simulink model "QBot2e_Forward_Kinematics"  (Simulink 8.9)
settings: Solver=ode1  StartTime=0.0  StopTime=inf  FixedStep=0.01  RelTol=1e-3  EnableMultiTasking=on
undefined symbols (not defined in the file or in its folder): HIL
libraries: quarc_library x7
settings Model: Creator=rhuq  LastModifiedBy=amolki  SimulationMode=external  ExtModeTrigDuration=10000
settings SolverCC: PositivePriorityOrder=on
settings OptimizationCC: ExpressionDepthLimit=2147483647  InitFltsAndDblsToZero=on  LifeSpan=auto
settings DebuggingCC: SaveWithParameterizedLinksMsg=none  SolverPrmCheckMsg=warning  ParameterPrecisionLossMsg=none
settings SFSimCC: SimParseCustomCode=off
settings RTWCC: SystemTargetFile=quarc_linux_pi_3.tlc  TemplateMakefile=quarc_linux_pi_3_tmf  Description=QUARC Linux Raspberry Pi 3 Target
settings STFCustomTargetCC: TargetLibSuffix=.a  TargetPreCompLibLocation=C:\PROGRA~3\QUARC\lib\2017a\LICFC8~1\release  ConcurrentExecutionCompliant=on  SystemTargetFile=quarc_linux_pi_3.tlc
settings GRTTargetCC: TargetLibSuffix=.a  TargetPreCompLibLocation=C:\PROGRA~3\QUARC\lib\2017a\LICFC8~1\release  ParMdlRefBuildCompliant=off  CompOptLevelCompliant=off  GeneratePreprocessorConditionals=Use local settings  MatFileLogging=off  CPPClassGenCompliant=off  UseToolchainInfoCompliant=off  ExtMode=on  ExtModeMexFile=quarc_comm  ExtModeMexArgs='-w -d /tmp -uri %u'

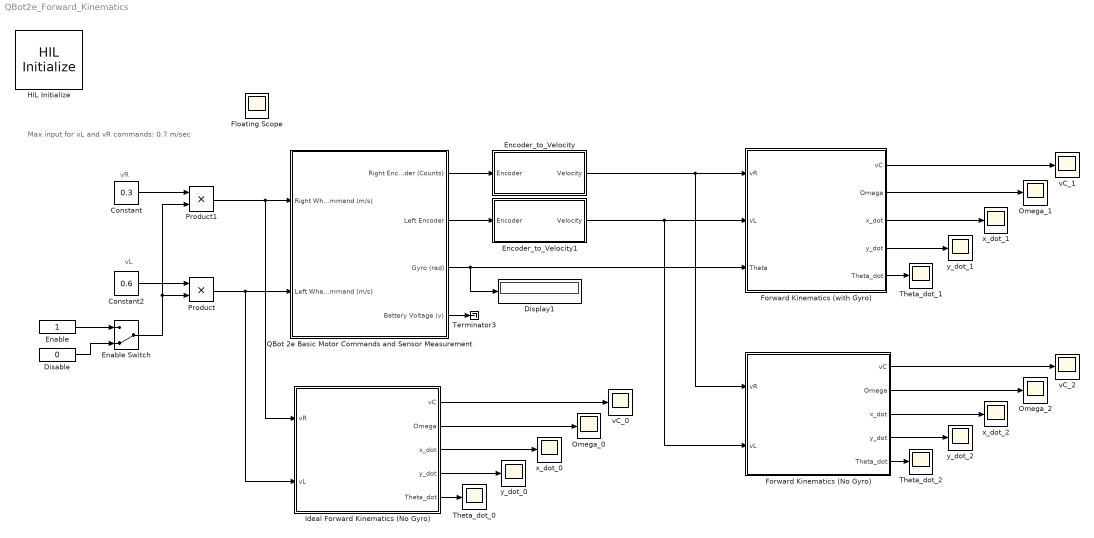
== system QBot2e_Forward_Kinematics ==
  note: vL
  note: vR
  note: Max input for vL and vR commands: 0.7 m/sec
  Constant : Constant  Value=0.3
  Constant2 : Constant  Value=0.6
  Disable : Constant  Value=0
  Display1 : Display
  Enable : Constant
  Enable Switch : ManualSwitch  CurrentSetting=0
  Encoder_to_Velocity : Subsystem
  Encoder_to_Velocity1 : Subsystem
  Forward Kinematics (No Gyro) : Subsystem
  Forward Kinematics (with Gyro) : Subsystem
  HIL Initialize : quarc_library/Data Acquisition/Generic/Configuration/HIL Initialize  Priority=-99  object_name=HIL-1  board_type=qbot2e  board_number=0  board_options=pwm0_en=1;pwm0_pin=12;pwm1_en=1;pwm1_pin=13;  exclusive=off  active=off  hardware_clocks=[]  clock_modes=[]  initial_clock_frequencies=[]  set_clock_params_at_start=off  set_clock_params_at_switch_in=off  set_clock_frequencies_at_start=off  set_clock_frequencies_at_switch_in=off  analog_input_channels=[0:5]  analog_input_configurations=[]  analog_input_maximums=[16.5 3.3 3.3 3.3 3.3 3.3]  analog_input_minimums=[0 0 0 0 0 0]  set_analog_input_params_at_start=off  set_analog_input_params_at_switch_in=off  analog_output_channels=[]  analog_output_maximums=[]  analog_output_minimums=[]  initial_analog_outputs=[]  final_analog_outputs=[]  watchdog_analog_outputs=[]  set_analog_output_params_at_start=off  set_analog_output_params_at_switch_in=off  set_analog_outputs_at_start=off  set_analog_outputs_at_switch_in=off  set_analog_outputs_at_terminate=off  set_analog_outputs_at_switch_out=off  set_analog_outputs_on_watchdog=off  digital_input_channels=[28:58]  digital_output_channels=[28:31]  digital_output_configuration=[]  initial_digital_outputs=[0]  final_digital_outputs=[0]  watchdog_digital_outputs=[]  set_digital_output_params_at_start=off  set_digital_output_params_at_switch_in=off  set_digital_outputs_at_start=on  set_digital_outputs_at_switch_in=off  set_digital_outputs_at_terminate=on  set_digital_outputs_at_switch_out=off  set_digital_outputs_on_watchdog=off  encoder_channels=[0:1]  quadrature=[4]  encoder_filter_frequency=[]  initial_encoder_counts=[0]  set_encoder_params_at_start=on  set_encoder_params_at_switch_in=off  set_encoder_counts_at_start=on  set_encoder_counts_at_switch_in=off  pwm_channels=[0:1]  pwm_modes=0  pwm_frequency=100e6 / 4095  pwm_configuration=[0]  pwm_alignment=[0]  pwm_polarity=[1]  pwm_leading_deadband=[]  pwm_trailing_deadband=[]  initial_pwm_outputs=[0]  final_pwm_outputs=[0]  watchdog_pwm_outputs=[]  set_pwm_params_at_start=on  set_pwm_params_at_switch_in=off  set_pwm_outputs_at_start=on  set_pwm_outputs_at_switch_in=off  set_pwm_outputs_at_terminate=on  set_pwm_outputs_at_switch_out=off  set_pwm_outputs_on_watchdog=off  other_output_channels=[2000:2001 14000 16000]  initial_other_outputs=[0 0 0 7]  final_other_outputs=[0 0 0 7]  watchdog_other_outputs=[]  set_other_outputs_at_start=on  set_other_outputs_at_switch_in=off  set_other_outputs_at_terminate=on  set_other_outputs_at_switch_out=off  set_other_outputs_on_watchdog=off
  Ideal Forward Kinematics (No Gyro) : Subsystem
  Omega_0 : Scope
  Omega_1 : Scope
  Omega_2 : Scope
  Product : Product  RndMeth=Zero
  Product1 : Product  RndMeth=Zero
  QBot 2e Basic Motor Commands and Sensor Measurement : Subsystem
  Terminator3 : Terminator
  Theta_dot_0 : Scope
  Theta_dot_1 : Scope
  Theta_dot_2 : Scope
  vC_0 : Scope
  vC_1 : Scope
  vC_2 : Scope
  x_dot_0 : Scope
  x_dot_1 : Scope
  x_dot_2 : Scope
  y_dot_0 : Scope
  y_dot_1 : Scope
  y_dot_2 : Scope
  Floating Scope : Scope
  wires:
  QBot 2e Basic Motor Commands and Sensor Measurement/1(Right Encoder (Counts)) -> Encoder_to_Velocity/1(Encoder)
  QBot 2e Basic Motor Commands and Sensor Measurement/2(Left Encoder) -> Encoder_to_Velocity1/1(Encoder)
  QBot 2e Basic Motor Commands and Sensor Measurement/3(Gyro (rad)) -> Display1/1, Forward Kinematics (with Gyro)/3(Theta)
  Encoder_to_Velocity1/1(Velocity) -> Forward Kinematics (No Gyro)/2(vL), Forward Kinematics (with Gyro)/2(vL)
  Ideal Forward Kinematics (No Gyro)/1(vC) -> vC_0/1
  Ideal Forward Kinematics (No Gyro)/2(Omega) -> Omega_0/1
  Encoder_to_Velocity/1(Velocity) -> Forward Kinematics (No Gyro)/1(vR), Forward Kinematics (with Gyro)/1(vR)
  Enable/1 -> Enable Switch/1
  Disable/1 -> Enable Switch/2
  Constant2/1 -> Product/1
  Constant/1 -> Product1/1
  Enable Switch/1 -> Product/2, Product1/2
  Product1/1 -> QBot 2e Basic Motor Commands and Sensor Measurement/1(Right Wheel Command (m/s)), Ideal Forward Kinematics (No Gyro)/1(vR)
  Product/1 -> Ideal Forward Kinematics (No Gyro)/2(vL), QBot 2e Basic Motor Commands and Sensor Measurement/2(Left Wheel Command (m/s))
  Ideal Forward Kinematics (No Gyro)/3(x_dot) -> x_dot_0/1
  Ideal Forward Kinematics (No Gyro)/4(y_dot) -> y_dot_0/1
  Ideal Forward Kinematics (No Gyro)/5(Theta_dot) -> Theta_dot_0/1
  Forward Kinematics (with Gyro)/1(vC) -> vC_1/1
  Forward Kinematics (with Gyro)/2(Omega) -> Omega_1/1
  Forward Kinematics (with Gyro)/3(x_dot) -> x_dot_1/1
  Forward Kinematics (with Gyro)/4(y_dot) -> y_dot_1/1
  Forward Kinematics (with Gyro)/5(Theta_dot) -> Theta_dot_1/1
  Forward Kinematics (No Gyro)/1(vC) -> vC_2/1
  Forward Kinematics (No Gyro)/2(Omega) -> Omega_2/1
  Forward Kinematics (No Gyro)/3(x_dot) -> x_dot_2/1
  Forward Kinematics (No Gyro)/4(y_dot) -> y_dot_2/1
  Forward Kinematics (No Gyro)/5(Theta_dot) -> Theta_dot_2/1
  QBot 2e Basic Motor Commands and Sensor Measurement/4(Battery Voltage (v)) -> Terminator3/1

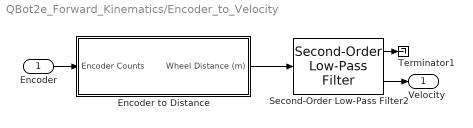
== system QBot2e_Forward_Kinematics/Encoder_to_Velocity ==
  Encoder : Inport
  Encoder to Distance : Subsystem
  Second-Order Low-Pass Filter2 : quarc_library/Continuous/Second-Order Low-Pass Filter  params_source=Internal (dialog parameters)  input_width=10  input_zeta=1  input_init=0
  Terminator1 : Terminator
  Velocity : Outport
  wires:
  Second-Order Low-Pass Filter2/2 -> Velocity/1
  Encoder/1 -> Encoder to Distance/1(Encoder Counts)
  Encoder to Distance/1(Wheel Distance (m)) -> Second-Order Low-Pass Filter2/1
  Second-Order Low-Pass Filter2/1 -> Terminator1/1

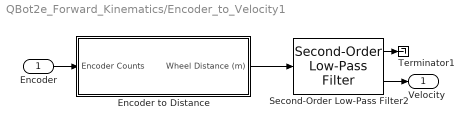
== system QBot2e_Forward_Kinematics/Encoder_to_Velocity1 ==
  Encoder : Inport
  Encoder to Distance : Subsystem
  Second-Order Low-Pass Filter2 : quarc_library/Continuous/Second-Order Low-Pass Filter  params_source=Internal (dialog parameters)  input_width=10  input_zeta=1  input_init=0
  Terminator1 : Terminator
  Velocity : Outport
  wires:
  Second-Order Low-Pass Filter2/2 -> Velocity/1
  Encoder/1 -> Encoder to Distance/1(Encoder Counts)
  Encoder to Distance/1(Wheel Distance (m)) -> Second-Order Low-Pass Filter2/1
  Second-Order Low-Pass Filter2/1 -> Terminator1/1

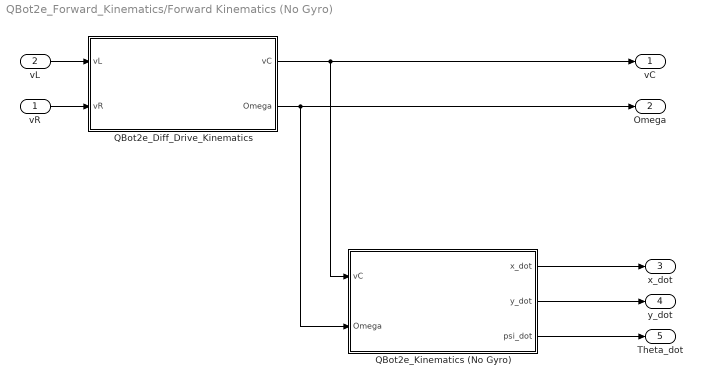
== system QBot2e_Forward_Kinematics/Forward Kinematics (No Gyro) ==
  vR : Inport
  vL : Inport  Port=2
  QBot2e_Diff_Drive_Kinematics : Subsystem
  QBot2e_Kinematics (No Gyro) : Subsystem
  vC : Outport
  Omega : Outport  Port=2
  x_dot : Outport  Port=3
  y_dot : Outport  Port=4
  Theta_dot : Outport  Port=5
  wires:
  QBot2e_Diff_Drive_Kinematics/2(Omega) -> QBot2e_Kinematics (No Gyro)/2(Omega), Omega/1
  vR/1 -> QBot2e_Diff_Drive_Kinematics/2(vR)
  vL/1 -> QBot2e_Diff_Drive_Kinematics/1(vL)
  QBot2e_Diff_Drive_Kinematics/1(vC) -> QBot2e_Kinematics (No Gyro)/1(vC), vC/1
  QBot2e_Kinematics (No Gyro)/2(y_dot) -> y_dot/1
  QBot2e_Kinematics (No Gyro)/1(x_dot) -> x_dot/1
  QBot2e_Kinematics (No Gyro)/3(psi_dot) -> Theta_dot/1

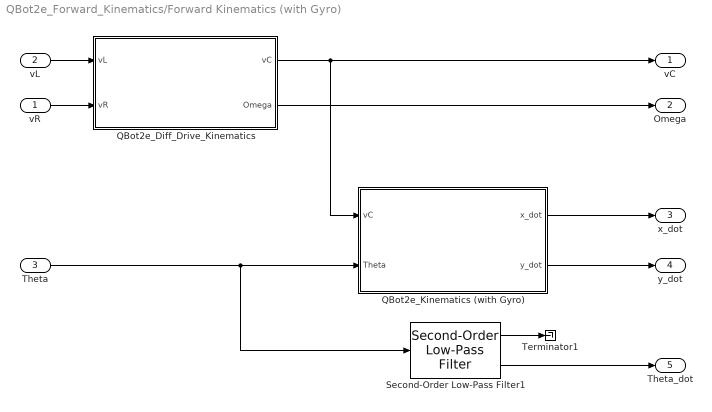
== system QBot2e_Forward_Kinematics/Forward Kinematics (with Gyro) ==
  vR : Inport
  vL : Inport  Port=2
  Theta : Inport  Port=3
  QBot2e_Diff_Drive_Kinematics : Subsystem
  QBot2e_Kinematics (with Gyro) : Subsystem
  Second-Order Low-Pass Filter1 : quarc_library/Continuous/Second-Order Low-Pass Filter  params_source=Internal (dialog parameters)  input_width=60  input_zeta=1  input_init=0
  Terminator1 : Terminator
  vC : Outport
  Omega : Outport  Port=2
  x_dot : Outport  Port=3
  y_dot : Outport  Port=4
  Theta_dot : Outport  Port=5
  wires:
  Second-Order Low-Pass Filter1/2 -> Theta_dot/1
  Second-Order Low-Pass Filter1/1 -> Terminator1/1
  QBot2e_Kinematics (with Gyro)/1(x_dot) -> x_dot/1
  QBot2e_Diff_Drive_Kinematics/1(vC) -> QBot2e_Kinematics (with Gyro)/1(vC), vC/1
  vL/1 -> QBot2e_Diff_Drive_Kinematics/1(vL)
  vR/1 -> QBot2e_Diff_Drive_Kinematics/2(vR)
  QBot2e_Diff_Drive_Kinematics/2(Omega) -> Omega/1
  QBot2e_Kinematics (with Gyro)/2(y_dot) -> y_dot/1
  Theta/1 -> QBot2e_Kinematics (with Gyro)/2(Theta), Second-Order Low-Pass Filter1/1

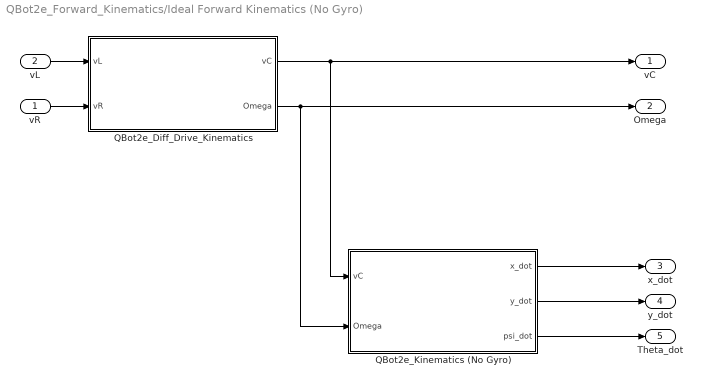
== system QBot2e_Forward_Kinematics/Ideal Forward Kinematics (No Gyro) ==
  vR : Inport
  vL : Inport  Port=2
  QBot2e_Diff_Drive_Kinematics : Subsystem
  QBot2e_Kinematics (No Gyro) : Subsystem
  vC : Outport
  Omega : Outport  Port=2
  x_dot : Outport  Port=3
  y_dot : Outport  Port=4
  Theta_dot : Outport  Port=5
  wires:
  QBot2e_Diff_Drive_Kinematics/2(Omega) -> QBot2e_Kinematics (No Gyro)/2(Omega), Omega/1
  vR/1 -> QBot2e_Diff_Drive_Kinematics/2(vR)
  vL/1 -> QBot2e_Diff_Drive_Kinematics/1(vL)
  QBot2e_Diff_Drive_Kinematics/1(vC) -> QBot2e_Kinematics (No Gyro)/1(vC), vC/1
  QBot2e_Kinematics (No Gyro)/2(y_dot) -> y_dot/1
  QBot2e_Kinematics (No Gyro)/1(x_dot) -> x_dot/1
  QBot2e_Kinematics (No Gyro)/3(psi_dot) -> Theta_dot/1

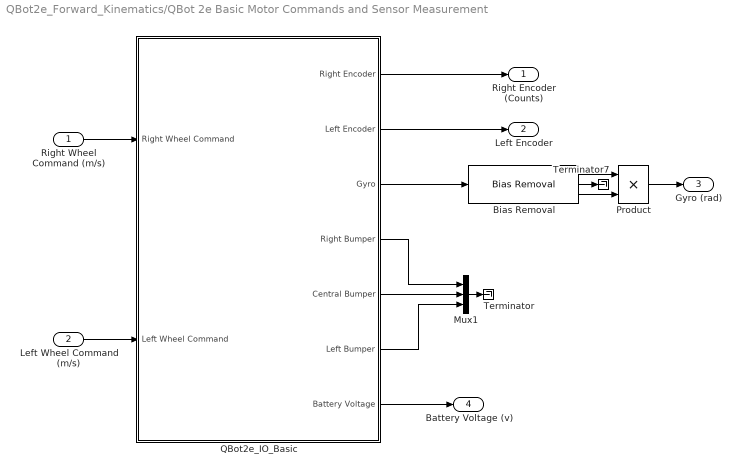
== system QBot2e_Forward_Kinematics/QBot 2e Basic Motor Commands and Sensor Measurement ==
  Right Wheel Command (m/s) : Inport
  Left Wheel Command (m/s) : Inport  Port=2
  Bias Removal : quarc_library/Discrete/Bias Removal  start_time=3  end_time=4  switch_id=0  sample_time=qc_get_step_size
      settings: SourceProductName=QUARC Targets
  Mux1 : Mux  Inputs=3
  Product : Product  RndMeth=Zero
  QBot2e_IO_Basic : Subsystem
  Terminator : Terminator
  Terminator7 : Terminator
  Right Encoder (Counts) : Outport
  Left Encoder : Outport  Port=2
  Gyro (rad) : Outport  Port=3
  Battery Voltage (v) : Outport  Port=4
  wires:
  QBot2e_IO_Basic/4(Right Bumper) -> Mux1/1
  QBot2e_IO_Basic/5(Central Bumper) -> Mux1/2
  QBot2e_IO_Basic/6(Left Bumper) -> Mux1/3
  Right Wheel Command (m/s)/1 -> QBot2e_IO_Basic/1(Right Wheel Command)
  Left Wheel Command (m/s)/1 -> QBot2e_IO_Basic/2(Left Wheel Command)
  QBot2e_IO_Basic/1(Right Encoder) -> Right Encoder (Counts)/1
  QBot2e_IO_Basic/2(Left Encoder) -> Left Encoder/1
  QBot2e_IO_Basic/7(Battery Voltage) -> Battery Voltage (v)/1
  Bias Removal/2 -> Terminator7/1
  Bias Removal/1 -> Product/1
  Bias Removal/3 -> Product/2
  Product/1 -> Gyro (rad)/1
  QBot2e_IO_Basic/3(Gyro) -> Bias Removal/1
  Mux1/1 -> Terminator/1

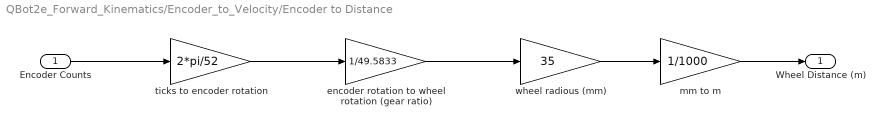
== system QBot2e_Forward_Kinematics/Encoder_to_Velocity/Encoder to Distance ==
  Encoder Counts : Inport
  " encoder rotation to wheel rotation (gear ratio)" : Gain  Gain=1/49.5833
  mm to m : Gain  Gain=1/1000
  ticks to encoder rotation : Gain  Gain=2*pi/52
  wheel radious (mm) : Gain  Gain=35
  Wheel Distance (m) : Outport
  wires:
  mm to m/1 -> Wheel Distance (m)/1
  wheel radious (mm)/1 -> mm to m/1
  " encoder rotation to wheel rotation (gear ratio)"/1 -> wheel radious (mm)/1
  ticks to encoder rotation/1 -> " encoder rotation to wheel rotation (gear ratio)"/1
  Encoder Counts/1 -> ticks to encoder rotation/1

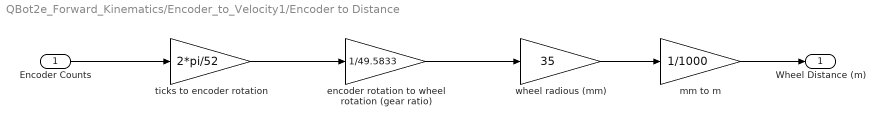
== system QBot2e_Forward_Kinematics/Encoder_to_Velocity1/Encoder to Distance ==
  Encoder Counts : Inport
  " encoder rotation to wheel rotation (gear ratio)" : Gain  Gain=1/49.5833
  mm to m : Gain  Gain=1/1000
  ticks to encoder rotation : Gain  Gain=2*pi/52
  wheel radious (mm) : Gain  Gain=35
  Wheel Distance (m) : Outport
  wires:
  mm to m/1 -> Wheel Distance (m)/1
  wheel radious (mm)/1 -> mm to m/1
  " encoder rotation to wheel rotation (gear ratio)"/1 -> wheel radious (mm)/1
  ticks to encoder rotation/1 -> " encoder rotation to wheel rotation (gear ratio)"/1
  Encoder Counts/1 -> ticks to encoder rotation/1

== system QBot2e_Forward_Kinematics/Forward Kinematics (No Gyro)/QBot2e_Diff_Drive_Kinematics ==
  vL : Inport
  vR : Inport  Port=2
  Qbot2_Diff_Drive_Kinematics : MATLAB Function  TreatAsAtomicUnit=on
  vC : Outport
  Omega : Outport  Port=2
  wires:
  vL/1 -> Qbot2_Diff_Drive_Kinematics/1(vL)
  Qbot2_Diff_Drive_Kinematics/1(vC) -> vC/1
  vR/1 -> Qbot2_Diff_Drive_Kinematics/2(vR)
  Qbot2_Diff_Drive_Kinematics/2(Omega) -> Omega/1

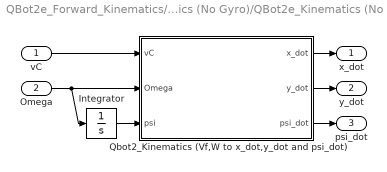
== system QBot2e_Forward_Kinematics/Forward Kinematics (No Gyro)/QBot2e_Kinematics (No Gyro) ==
  vC : Inport
  Omega : Inport  Port=2
  Integrator : Integrator
  Qbot2_Kinematics (Vf,W to x_dot,y_dot and psi_dot) : MATLAB Function  TreatAsAtomicUnit=on
  x_dot : Outport
  y_dot : Outport  Port=2
  psi_dot : Outport  Port=3
  wires:
  Qbot2_Kinematics (Vf,W to x_dot,y_dot and psi_dot)/3(psi_dot) -> psi_dot/1
  Integrator/1 -> Qbot2_Kinematics (Vf,W to x_dot,y_dot and psi_dot)/3(psi)
  vC/1 -> Qbot2_Kinematics (Vf,W to x_dot,y_dot and psi_dot)/1(vC)
  Qbot2_Kinematics (Vf,W to x_dot,y_dot and psi_dot)/1(x_dot) -> x_dot/1
  Omega/1 -> Integrator/1, Qbot2_Kinematics (Vf,W to x_dot,y_dot and psi_dot)/2(Omega)
  Qbot2_Kinematics (Vf,W to x_dot,y_dot and psi_dot)/2(y_dot) -> y_dot/1

== system QBot2e_Forward_Kinematics/Forward Kinematics (with Gyro)/QBot2e_Diff_Drive_Kinematics ==
  vL : Inport
  vR : Inport  Port=2
  Qbot2_Diff_Drive_Kinematics : MATLAB Function  TreatAsAtomicUnit=on
  vC : Outport
  Omega : Outport  Port=2
  wires:
  vL/1 -> Qbot2_Diff_Drive_Kinematics/1(vL)
  Qbot2_Diff_Drive_Kinematics/1(vC) -> vC/1
  vR/1 -> Qbot2_Diff_Drive_Kinematics/2(vR)
  Qbot2_Diff_Drive_Kinematics/2(Omega) -> Omega/1

== system QBot2e_Forward_Kinematics/Forward Kinematics (with Gyro)/QBot2e_Kinematics (with Gyro) ==
  vC : Inport
  Theta : Inport  Port=2
  Qbot2_Kinematics (Vf,W and Psi to x_dot,y_dot and psi_dot) : MATLAB Function  TreatAsAtomicUnit=on
  x_dot : Outport
  y_dot : Outport  Port=2
  wires:
  Theta/1 -> Qbot2_Kinematics (Vf,W and Psi to x_dot,y_dot and psi_dot)/2(psi)
  Qbot2_Kinematics (Vf,W and Psi to x_dot,y_dot and psi_dot)/2(y_dot) -> y_dot/1
  Qbot2_Kinematics (Vf,W and Psi to x_dot,y_dot and psi_dot)/1(x_dot) -> x_dot/1
  vC/1 -> Qbot2_Kinematics (Vf,W and Psi to x_dot,y_dot and psi_dot)/1(vC)

== system QBot2e_Forward_Kinematics/Ideal Forward Kinematics (No Gyro)/QBot2e_Diff_Drive_Kinematics ==
  vL : Inport
  vR : Inport  Port=2
  Qbot2_Diff_Drive_Kinematics : MATLAB Function  TreatAsAtomicUnit=on
  vC : Outport
  Omega : Outport  Port=2
  wires:
  vL/1 -> Qbot2_Diff_Drive_Kinematics/1(vL)
  Qbot2_Diff_Drive_Kinematics/1(vC) -> vC/1
  vR/1 -> Qbot2_Diff_Drive_Kinematics/2(vR)
  Qbot2_Diff_Drive_Kinematics/2(Omega) -> Omega/1

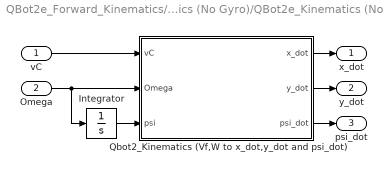
== system QBot2e_Forward_Kinematics/Ideal Forward Kinematics (No Gyro)/QBot2e_Kinematics (No Gyro) ==
  vC : Inport
  Omega : Inport  Port=2
  Integrator : Integrator
  Qbot2_Kinematics (Vf,W to x_dot,y_dot and psi_dot) : MATLAB Function  TreatAsAtomicUnit=on
  x_dot : Outport
  y_dot : Outport  Port=2
  psi_dot : Outport  Port=3
  wires:
  Qbot2_Kinematics (Vf,W to x_dot,y_dot and psi_dot)/3(psi_dot) -> psi_dot/1
  Integrator/1 -> Qbot2_Kinematics (Vf,W to x_dot,y_dot and psi_dot)/3(psi)
  vC/1 -> Qbot2_Kinematics (Vf,W to x_dot,y_dot and psi_dot)/1(vC)
  Qbot2_Kinematics (Vf,W to x_dot,y_dot and psi_dot)/1(x_dot) -> x_dot/1
  Omega/1 -> Integrator/1, Qbot2_Kinematics (Vf,W to x_dot,y_dot and psi_dot)/2(Omega)
  Qbot2_Kinematics (Vf,W to x_dot,y_dot and psi_dot)/2(y_dot) -> y_dot/1

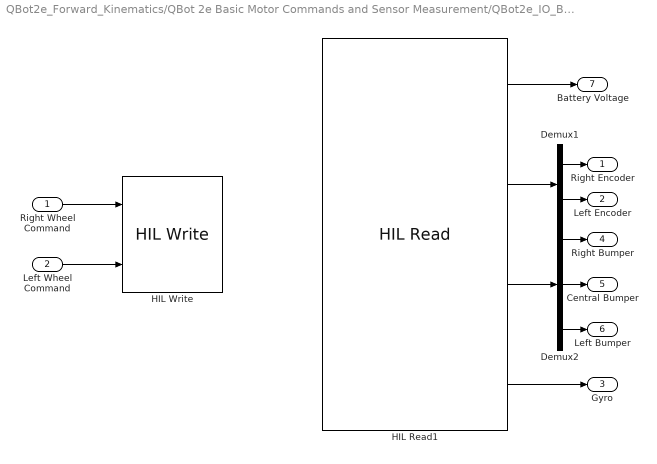
== system QBot2e_Forward_Kinematics/QBot 2e Basic Motor Commands and Sensor Measurement/QBot2e_IO_Basic ==
  Right Wheel Command : Inport
  Left Wheel Command : Inport  Port=2
  Demux1 : Demux  Outputs=2
  Demux2 : Demux  Outputs=3
  HIL Read1 : quarc_library/Data Acquisition/Generic/Immediate I//O/HIL Read  object_name=HIL-1  analog_channels=[0]  encoder_channels=[0:1]  digital_channels=[28:30]  other_channels=[1002]  sample_time=qc_get_step_size  active=on  vector_output=on  data_type_mode=Inherit via back propagation  encoder_data_type=double  digital_data_type=boolean
  HIL Write : quarc_library/Data Acquisition/Generic/Immediate I//O/HIL Write  object_name=HIL-1  analog_channels=[]  pwm_channels=[]  digital_channels=[]  other_channels=[2000:2001]  sample_time=-1  active=on  vector_input=off
  Right Encoder : Outport
  Left Encoder : Outport  Port=2
  Gyro : Outport  Port=3
  Right Bumper : Outport  Port=4
  Central Bumper : Outport  Port=5
  Left Bumper : Outport  Port=6
  Battery Voltage : Outport  Port=7
  wires:
  HIL Read1/1 -> Battery Voltage/1
  HIL Read1/3 -> Demux2/1
  HIL Read1/4 -> Gyro/1
  Demux1/1 -> Right Encoder/1
  Demux1/2 -> Left Encoder/1
  Right Wheel Command/1 -> HIL Write/1
  Left Wheel Command/1 -> HIL Write/2
  HIL Read1/2 -> Demux1/1
  Demux2/1 -> Right Bumper/1
  Demux2/2 -> Central Bumper/1
  Demux2/3 -> Left Bumper/1

== matlab function Forward Kinematics (No Gyro)/QBot2e_Diff_Drive_Kinematics/Qbot2_Diff_Drive_Kinematics ==
  data: vL input double; vC output double; vR input double; Omega output double
function [vC,Omega] = fcn(vL,vR)
%#codegen

d= 0.235;

vC=0.5*(vL+vR);
Omega=(1/d)*(vR-vL);

== matlab function Forward Kinematics (with Gyro)/QBot2e_Diff_Drive_Kinematics/Qbot2_Diff_Drive_Kinematics ==
  data: vL input double; vC output double; vR input double; Omega output double
function [vC,Omega] = fcn(vL,vR)
%#codegen

d= 0.235;

vC=0.5*(vL+vR);
Omega=(1/d)*(vR-vL);

== matlab function Forward Kinematics (with Gyro)/QBot2e_Kinematics (with Gyro)/Qbot2_Kinematics (Vf,W and Psi to x_dot,y_dot and psi_dot) ==
  data: vC input double; x_dot output double; y_dot output double; psi input double
function [x_dot,y_dot] = fcn(vC,psi)
%#codegen


x_dot=cos(psi)*vC;
y_dot=sin(psi)*vC;

== matlab function Forward Kinematics (No Gyro)/QBot2e_Kinematics (No Gyro)/Qbot2_Kinematics (Vf,W to x_dot,y_dot and psi_dot) ==
  data: vC input double; x_dot output double; Omega input double; y_dot output double; psi input double; psi_dot output double
function [x_dot,y_dot,psi_dot] = fcn(vC,Omega,psi)
%#codegen


x_dot=cos(psi)*vC;
y_dot=sin(psi)*vC;
psi_dot= Omega;

== matlab function Ideal Forward Kinematics (No Gyro)/QBot2e_Diff_Drive_Kinematics/Qbot2_Diff_Drive_Kinematics ==
  data: vL input double; vC output double; vR input double; Omega output double
function [vC,Omega] = fcn(vL,vR)
%#codegen

d= 0.235;

vC=0.5*(vL+vR);
Omega=(1/d)*(vR-vL);

== matlab function Ideal Forward Kinematics (No Gyro)/QBot2e_Kinematics (No Gyro)/Qbot2_Kinematics (Vf,W to x_dot,y_dot and psi_dot) ==
  data: vC input double; x_dot output double; Omega input double; y_dot output double; psi input double; psi_dot output double
function [x_dot,y_dot,psi_dot] = fcn(vC,Omega,psi)
%#codegen


x_dot=cos(psi)*vC;
y_dot=sin(psi)*vC;
psi_dot= Omega;
